simulink model "Sigi_SISO_LQR_Fullstate_stabilisiert"  (R2019a)
settings: Solver=ode4  StartTime=0.0  StopTime=par.t_sim  FixedStep=par.Ts  MaxStep=1e-5  RelTol=1e-3
values from neighbouring files (symbols this model uses):
  d_p_0 = 0    [01_Sigi_v2_LQR_Design.m]
  d_theta_0 = 0    [01_Sigi_v2_LQR_Design.m]
  K_lqr = lqr(A,B,Q,R)    [Design_LQR_3x3.m]    (also in Design_LQR_Fullstate.m; Sigi_SISO_LQR_3x3_stabilisiert_NonlinearODE.m = [K_lqr_1, K_lqr_2, K_lqr_3]; Sigi_SISO_LQR_Fullstate_stabilisiert_NonlinearODE.m = [K_lqr_1, K_lqr_2, K_lqr_3, K_lqr_4])
  p_0 = 0    [01_Sigi_v2_LQR_Design.m]
  theta_0 = -25 /360*2*pi    (= -0.436332312999)    [01_Sigi_v2_LQR_Design.m]
undefined symbols (not defined in the file or in its folder): par
settings Model: Creator=Raffi  LastModifiedBy=Raffi
settings ModelReferenceCC: ModelReferenceMinAlgLoopOccurrences=on

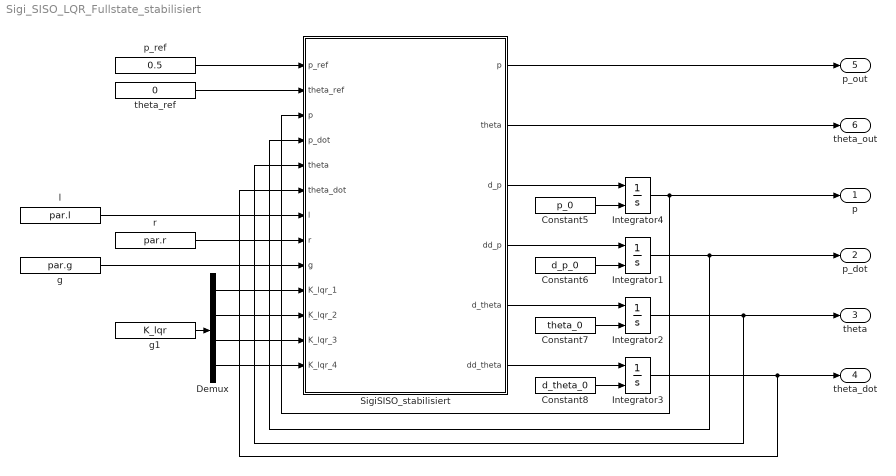
== system Sigi_SISO_LQR_Fullstate_stabilisiert ==
  Constant5 : Constant  Value=p_0
  Constant6 : Constant  Value=d_p_0
  Constant7 : Constant  Value=theta_0
  Constant8 : Constant  Value=d_theta_0
  Demux : Demux
  Integrator{1..4} (4 alike) : Integrator  InitialConditionSource=external
  SigiSISO_stabilisiert : MATLAB Function  TreatAsAtomicUnit=on
  g : Constant  Value=par.g
  g1 : Constant  Value=K_lqr
  l : Constant  Value=par.l
  p_ref : Constant  Value=0.5
  r : Constant  Value=par.r
  theta_ref : Constant  Value=0
  p : Outport
  p_dot : Outport  Port=2
  theta : Outport  Port=3
  theta_dot : Outport  Port=4
  p_out : Outport  Port=5
  theta_out : Outport  Port=6
  wires:
  SigiSISO_stabilisiert/5(d_theta) -> Integrator2/1
  SigiSISO_stabilisiert/6(dd_theta) -> Integrator3/1
  r/1 -> SigiSISO_stabilisiert/8(r)
  g/1 -> SigiSISO_stabilisiert/9(g)
  SigiSISO_stabilisiert/3(d_p) -> Integrator4/1
  Constant7/1 -> Integrator2/2
  Constant8/1 -> Integrator3/2
  Constant6/1 -> Integrator1/2
  Constant5/1 -> Integrator4/2
  SigiSISO_stabilisiert/4(dd_p) -> Integrator1/1
  Integrator4/1 -> p/1, SigiSISO_stabilisiert/3("p ")
  Integrator3/1 -> theta_dot/1, SigiSISO_stabilisiert/6(theta_dot)
  SigiSISO_stabilisiert/1(p) -> p_out/1
  l/1 -> SigiSISO_stabilisiert/7(l)
  SigiSISO_stabilisiert/2(theta) -> theta_out/1
  Integrator1/1 -> p_dot/1, SigiSISO_stabilisiert/4(p_dot)
  Integrator2/1 -> SigiSISO_stabilisiert/5("theta "), theta/1
  theta_ref/1 -> SigiSISO_stabilisiert/2(theta_ref)
  p_ref/1 -> SigiSISO_stabilisiert/1(p_ref)
  g1/1 -> Demux/1
  Demux/4 -> SigiSISO_stabilisiert/13(K_lqr_4)
  Demux/3 -> SigiSISO_stabilisiert/12(K_lqr_3)
  Demux/2 -> SigiSISO_stabilisiert/11(K_lqr_2)
  Demux/1 -> SigiSISO_stabilisiert/10(K_lqr_1)

== matlab function Sigi_SISO_LQR_Fullstate_stabilisiert/SigiSISO_stabilisiert ==
  data: p_ref input; theta_ref input; p output; theta output; p input; d_p output; p_dot input; theta input; theta_dot input; dd_p output; d_theta output; dd_theta output; l input; r input; g input; K_lqr_1 input; K_lqr_2 input; K_lqr_3 input; K_lqr_4 input
% This embedded Matlab function is only used to simulate an external Matlab
% function stored in a .m-file.
function [p,theta,...                               % Sytem outputs
    d_p,dd_p,d_theta,dd_theta] = ...                % State updates
    SigiSISO_stabilisiert(...
    p_ref, theta_ref,...                                   % Sytem input
    p,p_dot,theta,theta_dot,...                     % System states
    l, r, g,...                                     % System parameters
    K_lqr_1, K_lqr_2, K_lqr_3, K_lqr_4)                                         % LQR controller

% Run external Matlab function
    [p,theta,...                                    % Sytem outputs
    d_p,dd_p,d_theta,dd_theta] = ...                % State updates
    Sigi_SISO_LQR_Fullstate_stabilisiert_NonlinearODE(...
    p_ref, theta_ref,...                                   % Sytem input
    p,p_dot,theta,theta_dot,...                     % System states
    l, r, g,...                                     % System parameters
    K_lqr_1, K_lqr_2, K_lqr_3, K_lqr_4);                                         % LQR controller
